simulink model "frame_ctrl_test"  (R2021b)
settings: Solver=VariableStepAuto  StartTime=0.0  StopTime=stop_time-1  RelTol=1e-3
libraries: dspsrcs4 x1
settings Model: Creator=torha  LastModifiedBy=torha
settings SolverCC: AlgebraicLoopSolver=TrustRegion
settings DebuggingCC: SFMachineParentedDataDiag=warning

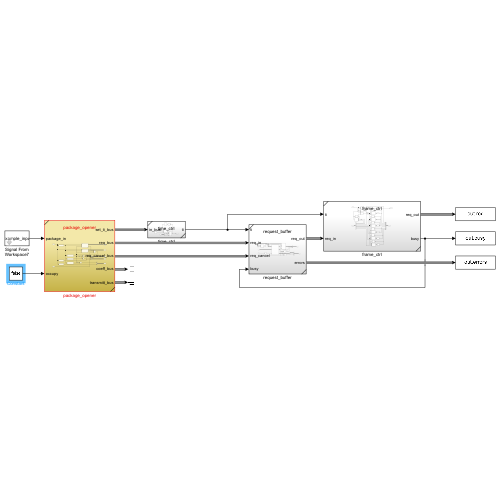
[thumbnail: Simulink's stored preview of the top-level diagram]
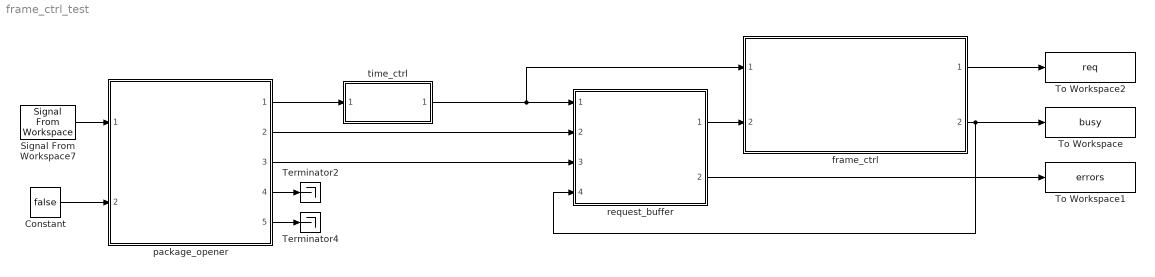
== system frame_ctrl_test ==
  Constant : Constant  Value=false
  Signal From Workspace7 : dspsrcs4/Signal From Workspace  X=example_input  Ts=1  nsamps=1  OutputAfterFinalValue=Setting to zero  ignoreOrWarnInputAndFrameLengths=off  OutputFrames=off
  Terminator2 : Terminator
  Terminator4 : Terminator
  To Workspace : ToWorkspace  VariableName=busy  SampleTime=-1
      settings: Save2DSignal=2-D array (concatenate along first dimension)
  To Workspace1 : ToWorkspace  VariableName=errors  SaveFormat=Timeseries  SampleTime=-1
  To Workspace2 : ToWorkspace  VariableName=req  SaveFormat=Timeseries  SampleTime=-1
  frame_ctrl : Subsystem  ReferencedSubsystem=frame_ctrl
  package_opener : Subsystem  ReferencedSubsystem=package_opener
  request_buffer : Subsystem  ReferencedSubsystem=request_buffer
  time_ctrl : Subsystem  ReferencedSubsystem=time_ctrl
  wires:
  frame_ctrl/2 -> request_buffer/4, To Workspace/1
  frame_ctrl/1 -> To Workspace2/1
  package_opener/1 -> time_ctrl/1
  package_opener/3 -> request_buffer/3
  Signal From Workspace7/1 -> package_opener/1
  request_buffer/2 -> To Workspace1/1
  request_buffer/1 -> frame_ctrl/2
  package_opener/5 -> Terminator4/1
  package_opener/4 -> Terminator2/1
  package_opener/2 -> request_buffer/2
  time_ctrl/1 -> request_buffer/1, frame_ctrl/1
  Constant/1 -> package_opener/2
